simulink model "linear_model"  (R2024a)
settings: Solver=VariableStepAuto  StartTime=0.0  StopTime=10.0  RelTol=1e-3
undefined symbols (not defined in the file or in its folder): f0, J, Kb, Kt, La, Ra
settings Model: Creator=rajam  LastModifiedBy=114121117

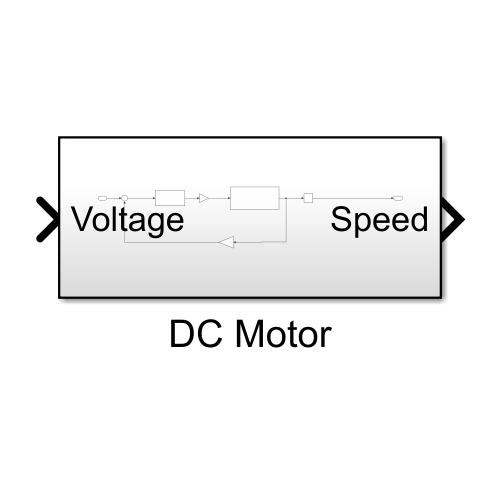
[thumbnail: Simulink's stored preview of the top-level diagram]
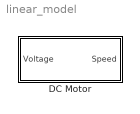
== system linear_model ==
  DC Motor : Subsystem

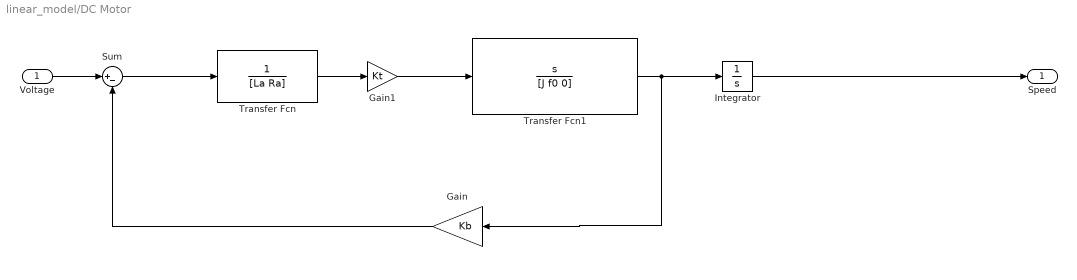
== system linear_model/DC Motor ==
  Voltage : Inport
  Gain : Gain  Gain=Kb
  Gain1 : Gain  Gain=Kt
  Integrator : Integrator
  Sum : Sum  Inputs=|+-
  Transfer Fcn : TransferFcn  Denominator=[La Ra]
  Transfer Fcn1 : TransferFcn  Numerator=[1 0]  Denominator=[J f0 0]
  Speed : Outport
  wires:
  Voltage/1 -> Sum/1
  Sum/1 -> Transfer Fcn/1
  Transfer Fcn/1 -> Gain1/1
  Gain1/1 -> Transfer Fcn1/1
  Transfer Fcn1/1 -> Integrator/1, Gain/1
  Gain/1 -> Sum/2
  Integrator/1 -> Speed/1
